simulink model "cartPend_MPC"  (R2023b)
settings: Solver=ode4  StartTime=0.0  StopTime=5  FixedStep=0.001  RelTol=1e-3
values from neighbouring files (symbols this model uses):
  Fc = 0.00040    (= 0.0004)    [MPC_casadi_block.m]    (also in continuous_cartpend.m; init_HAC_simulation.m; init_MPC.m; init_NMPC.m)
  g = [g; st_next - st_next_RK4]    [MPC_cartPend_casadi.m]    (also in MPC_cartPend_casadi_scaled.m; MPC_casadi_block.m; continuous_cartpend.m = 9.80665; init_HAC_simulation.m = 9.80665)
  I = 8.7395e-04    (= 0.00087395)    [MPC_casadi_block.m]    (also in continuous_cartpend.m = 0.0008739525; init_HAC_simulation.m = 0.0008739525; init_MPC.m = 0.0008739525; init_NMPC.m = 0.0008739525)
  init_angle = 180    [MPC_cartPend_casadi.m]    (also in init_HAC_simulation.m = 0.349065850399; init_MPC.m = -0.349065850399; init_NMPC.m = 3.14159265359; init_PID_cartpole.m = 0)
  kd = 0.000161    [MPC_casadi_block.m]    (also in continuous_cartpend.m; init_HAC_simulation.m; init_MPC.m; init_NMPC.m)
  kdr = 0.000001    (= 1e-06)    [MPC_casadi_block.m]    (also in continuous_cartpend.m; init_HAC_simulation.m; init_MPC.m; init_NMPC.m)
  kt = 150    [MPC_casadi_block.m]    (also in continuous_cartpend.m; init_HAC_simulation.m; init_MPC.m; init_NMPC.m)
  L = 0.1500    (= 0.15)    [MPC_casadi_block.m]    (also in continuous_cartpend.m; init_HAC_simulation.m; init_MPC.m; init_NMPC.m)
  m = 0.116527    [MPC_casadi_block.m]    (also in continuous_cartpend.m; init_HAC_simulation.m; init_MPC.m; init_NMPC.m)
  X0 = [X0(2:end,:);X0(end,:)]    [MPC_cartPend_casadi.m]    (also in MPC_cartPend_casadi_scaled.m; MPC_casadi_block.m = repmat(X, 1, obj.N+1); init_NMPC.m = [0; 0; init_angle; 0])
libraries: simulink_extras x2
settings Model: Creator=doann  LastModifiedBy=doann
settings OptimizationCC: DefaultParameterBehavior=Inlined  UseDivisionForNetSlopeComputation=on  GainParamInheritBuiltInType=on  UseFloatMulNetSlope=on  InlineInvariantSignals=on  ReuseModelBlockBuffer=off  PassReuseOutputArgsAs=Individual arguments  ZeroExternalMemoryAtStartup=off  ZeroInternalMemoryAtStartup=off  NoFixptDivByZeroProtection=on  EfficientFloat2IntCast=on  LifeSpan=1  OptimizeBlockOrder=speed  DifferentSizesBufferReuse=on  EfficientTunableParamExpr=on
settings DebuggingCC: ParameterTunabilityLossMsg=error
settings HardwareCC: ProdBitPerPointer=32  ProdBitPerSizeT=32  ProdBitPerPtrDiffT=32  ProdLargestAtomicInteger=Long  ProdLargestAtomicFloat=Double  ProdWordSize=32  ProdLongLongMode=on  ProdHWDeviceType=ARM Compatible->ARM Cortex-M
settings SFSimCC: MATLABDynamicMemAlloc=off
settings RTWCC: Description=Embedded Coder  SystemTargetFile=ert.tlc  TemplateMakefile=ert_default_tmf  TargetLang=C++
settings CodeAppCC: ForceParamTrailComments=on  IgnoreCustomStorageClasses=off  OperatorAnnotations=on  SimulinkDataObjDesc=on  SFDataObjDesc=on  CustomSymbolStrGlobalVar=rt$N$M  CustomSymbolStrType=$N$M  CustomSymbolStrFcn=$N$M$F  CustomSymbolStrMacro=$N$M  InsertBlockDesc=on
settings ERTTargetCC: TargetLangStandard=C++11 (ISO)  GenerateSampleERTMain=on  IncludeMdlTerminateFcn=off  CombineSignalStateStructs=on  SupportAbsoluteTime=off  CodeInterfacePackaging=C++ class  SupportComplex=off  SupportContinuousTime=on  SupportNonInlinedSFcns=on  InlinedParameterPlacement=NonHierarchical  RootIOFormat=Structure reference  ERTCustomFileTemplate=example_file_process.tlc  ERTFilePackagingFormat=CompactWithDataFile

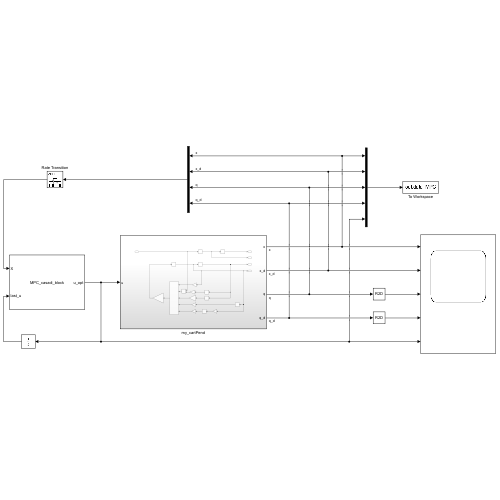
[thumbnail: Simulink's stored preview of the top-level diagram]
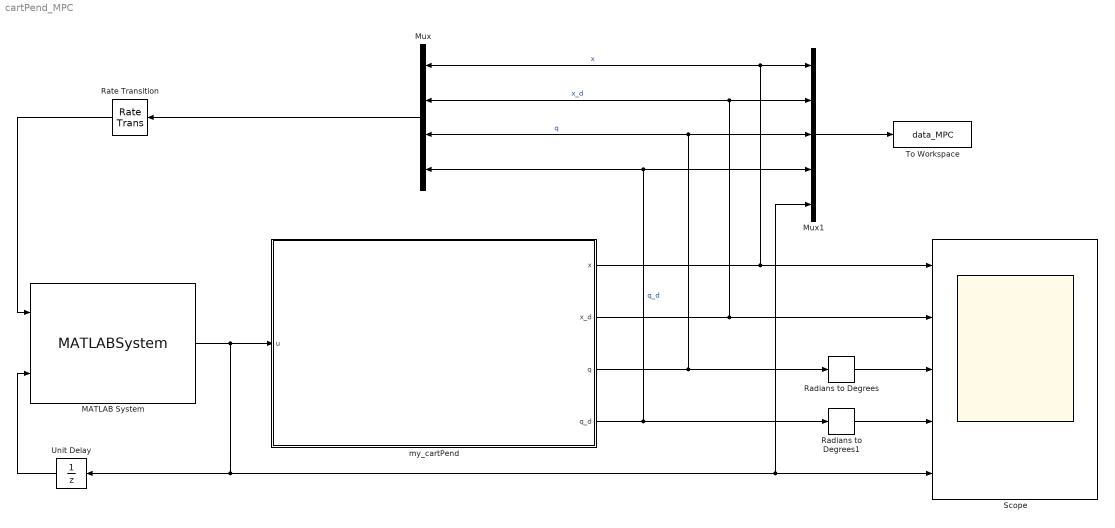
== system cartPend_MPC ==
  MATLAB System : MATLABSystem  System=MPC_casadi_block  T=0.1  N=15  Q=diag( [ 3, 0, 3, 0 ] )  R=0.01  xs=[ 0; 0; 0; 0 ]  SimulateUsing=Interpreted execution
      mask Type: MPC_casadi_block
      mask Display:
      | disp('MPC_casadi_block');
      | port_label('input',1,'X');
      | port_label('input',2,'last_u');
      | port_label('output',1,'u_opt');
  Mux : Mux
  Mux1 : Mux  Inputs=5
  Radians to Degrees : simulink_extras/Transformations/Radians to Degrees
  Radians to Degrees1 : simulink_extras/Transformations/Radians to Degrees
  Rate Transition : RateTransition  InitialCondition=X0  OutPortSampleTime=0.1
  Scope : Scope  NumInputPorts=5
  To Workspace : ToWorkspace  VariableName=data_MPC  SaveFormat=Timeseries  SampleTime=-1
  Unit Delay : UnitDelay  SampleTime=0.1  HasFrameUpgradeWarning=on
  my_cartPend : Subsystem
  wires:
  my_cartPend/1(x) -> Mux/1, Mux1/1, Scope/1  "x"
  my_cartPend/2(x_d) -> Mux/2, Mux1/2, Scope/2  "x_d"
  my_cartPend/3(q) -> Mux1/3, Mux/3, Radians to Degrees/1  "q"
  my_cartPend/4(q_d) -> Mux/4, Mux1/4, Radians to Degrees1/1  "q_d"
  Radians to Degrees/1 -> Scope/3
  Radians to Degrees1/1 -> Scope/4
  MATLAB System/1 -> Unit Delay/1, Mux1/5, Scope/5, my_cartPend/1(u)
  Mux/1 -> Rate Transition/1
  Mux1/1 -> To Workspace/1
  Rate Transition/1 -> MATLAB System/1
  Unit Delay/1 -> MATLAB System/2

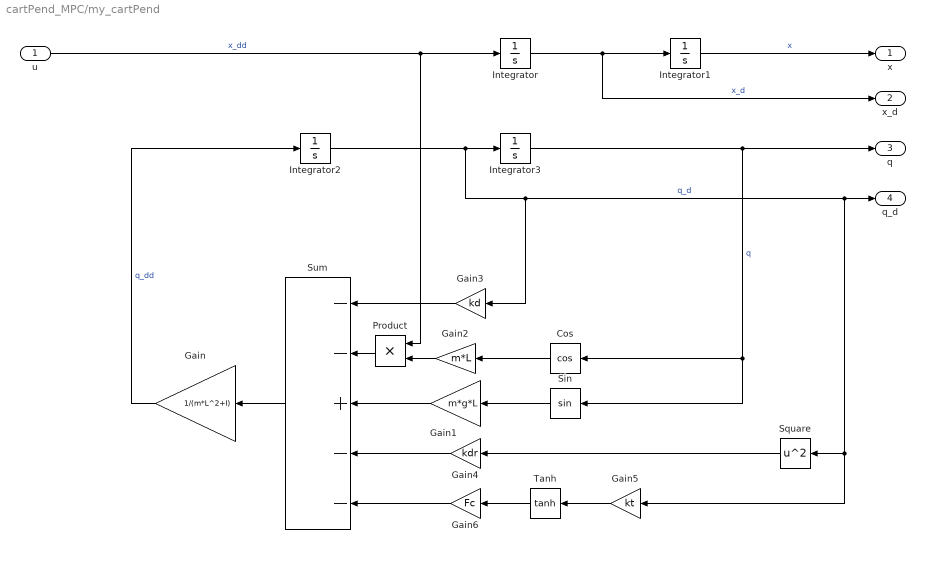
== system cartPend_MPC/my_cartPend ==
  u : Inport
  Cos : Trigonometry  Operator=cos
  Gain : Gain  Gain=1/(m*L^2+I)
  Gain1 : Gain  Gain=m*g*L
  Gain2 : Gain  Gain=m*L
  Gain3 : Gain  Gain=kd
  Gain4 : Gain  Gain=kdr
  Gain5 : Gain  Gain=kt
  Gain6 : Gain  Gain=Fc
  Integrator : Integrator
  Integrator1 : Integrator
  Integrator2 : Integrator
  Integrator3 : Integrator  InitialCondition=init_angle
  Product : Product
  Sin : Trigonometry
  Square : Math  Operator=square
  Sum : Sum  Inputs=--+--
  Tanh : Trigonometry  Operator=tanh
  x : Outport
  x_d : Outport  Port=2
  q : Outport  Port=3
  q_d : Outport  Port=4
  wires:
  u/1 -> Product/1, Integrator/1  "x_dd"
  Integrator/1 -> x_d/1, Integrator1/1  "x_d"
  Integrator1/1 -> x/1  "x"
  Integrator3/1 -> Sin/1, Cos/1, q/1  "q"
  Integrator2/1 -> Gain3/1, Gain5/1, Square/1, q_d/1, Integrator3/1  "q_d"
  Sin/1 -> Gain1/1
  Cos/1 -> Gain2/1
  Sum/1 -> Gain/1
  Gain/1 -> Integrator2/1  "q_dd"
  Gain1/1 -> Sum/3
  Gain3/1 -> Sum/1
  Gain2/1 -> Product/2
  Product/1 -> Sum/2
  Square/1 -> Gain4/1
  Tanh/1 -> Gain6/1
  Gain5/1 -> Tanh/1
  Gain4/1 -> Sum/4
  Gain6/1 -> Sum/5
